simulink library "BdyFrameGravForce_ul"  (R2018b)
settings: Solver=VariableStepAuto  StartTime=0.0  StopTime=10.0  RelTol=1e-3
undefined symbols (not defined in the file): gravAcc, massBdy
libraries: eulAng2RotMat_ul x1
settings Model: Creator=Ayaz  LastModifiedBy=asiddiq2

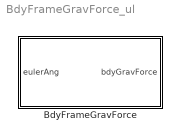
== system BdyFrameGravForce_ul ==
  BdyFrameGravForce : Subsystem  mask{gravAcc=gravAcc, massBdy=massBdy}
      mask prompts: gravAcc "Gravitational acceleration"; massBdy "Mass"
      mask DialogControl ParameterGroupVar Prompt: Environment
      mask DialogControl Container3 Prompt: Vehicle

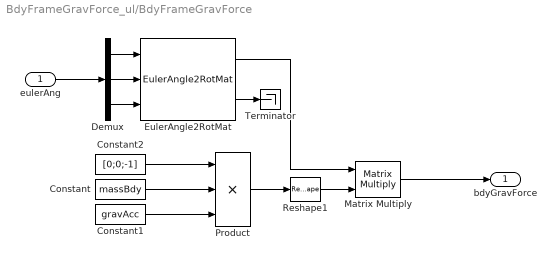
== system BdyFrameGravForce_ul/BdyFrameGravForce ==
  eulerAng : Inport  PortDimensions=[3,1]
  Constant : Constant  Value=massBdy  VectorParams1D=off
  Constant1 : Constant  Value=gravAcc  VectorParams1D=off
  Constant2 : Constant  Value=[0;0;-1]  VectorParams1D=off
  Demux : Demux  Outputs=3
  EulerAngle2RotMat : eulAng2RotMat_ul/EulerAngle2RotMat  SystemSampleTime=-1
  Matrix Multiply : Product  Multiplication=Matrix(*)
  Product : Product  Inputs=3
  Reshape1 : Reshape  OutputDimensionality=Column vector (2-D)
  Terminator : Terminator
  bdyGravForce : Outport  PortDimensions=[3,1]
  wires:
  eulerAng/1 -> Demux/1
  Demux/1 -> EulerAngle2RotMat/1
  Demux/2 -> EulerAngle2RotMat/2
  Demux/3 -> EulerAngle2RotMat/3
  Constant1/1 -> Product/3
  Constant2/1 -> Product/1
  EulerAngle2RotMat/2 -> Terminator/1
  Product/1 -> Reshape1/1
  EulerAngle2RotMat/1 -> Matrix Multiply/1
  Reshape1/1 -> Matrix Multiply/2
  Matrix Multiply/1 -> bdyGravForce/1
  Constant/1 -> Product/2
